simulink model "datatypedemo"  (Simulink 6.0)
settings: Solver=FixedStepDiscrete  SolverMode=SingleTasking  StartTime=0.0  StopTime=4  FixedStep=.01  RelTol=1e-3
settings Model: Creator=The MathWorks Inc.  LastModifiedBy=batserve  ExtModeTrigMode=oneshot  ExtModeArmWhenConnect=off  ExtModeAutoUpdateStatusClock=off
settings DataIOCC: LimitDataPoints=off
settings OptimizationCC: BooleanDataType=off
settings DebuggingCC: CheckExecutionContextPreStartOutputMsg=on  CheckExecutionContextRuntimeOutputMsg=on  SolverPrmCheckMsg=none  IntegerOverflowMsg=none
settings HardwareCC: TargetUnknown=on

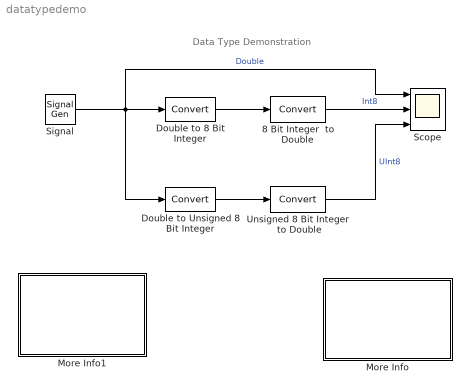
== system datatypedemo ==
  note: Data Type Demonstration
  8 Bit Integer  to Double : DataTypeConversion  OutDataTypeMode=double  SaturateOnIntegerOverflow=on  RndMeth=Zero
  Double to 8 Bit Integer : DataTypeConversion  OutDataTypeMode=int8  SaturateOnIntegerOverflow=on  RndMeth=Zero
  Double to Unsigned 8 Bit Integer : DataTypeConversion  OutDataTypeMode=uint8  SaturateOnIntegerOverflow=on  RndMeth=Zero
  More Info : Subsystem  PropExecContextAcrossSSBoundary=on
      mask Display: disp('Double click\nhere for\ninformation on\nthis demonstration')
  More Info1 : Subsystem  PropExecContextAcrossSSBoundary=on
      settings: OpenFcn=simcad(bdroot);
      mask Display: disp('Double click\nhere for\nSimulink Help')
  Scope : Scope  NumInputPorts=3
      settings: StartFcn=open_system(gcbh)  TimeRange=4  YMin=-150~-150~-150  YMax=150~150~150  DataFormat=Array
  Signal : SignalGenerator  Amplitude=150
      settings: AttributesFormatString=Waveform: %<Waveform>\nAmplitude: %<Amplitude>\nFreq: %<Frequency> %<Units>
  Unsigned 8 Bit Integer  to Double : DataTypeConversion  OutDataTypeMode=double  SaturateOnIntegerOverflow=on  RndMeth=Zero
  wires:
  Double to 8 Bit Integer/1 -> 8 Bit Integer  to Double/1
  8 Bit Integer  to Double/1 -> Scope/2  "Int8"
  Signal/1 -> Double to 8 Bit Integer/1, Scope/1, Double to Unsigned 8 Bit Integer/1  "Double"
  Unsigned 8 Bit Integer  to Double/1 -> Scope/3  "UInt8"
  Double to Unsigned 8 Bit Integer/1 -> Unsigned 8 Bit Integer  to Double/1

== system datatypedemo/More Info ==
  note: This demonstration shows how to use data types in Simulink.  For this simple
      | example, a sine wave with an amplitude of 150 is kept as a double, converted to
      | an 8-bit integer and converted to an unsigned 8-bit integer.  The resulting effects
      | of this are shown on a scope.  Notice that the signed integer is allowed to be
      | positive and negative but gets saturated above 128.  The unsigned integer is always
      | positive but does not get saturated until 256.
  note: Data Type Demonstration

== system datatypedemo/More Info1 ==
